simulink model "inverted"  (R2023b)
settings: Solver=VariableStepAuto  StartTime=0.0  StopTime=10.0  RelTol=1e-3
values from neighbouring files (symbols this model uses):
  A = [0 1 0 0 ... (first row only)    [invertedpendulum.m]
  B = [0 ... (first row only)    [invertedpendulum.m]
  C = [0 0 1 0]    [invertedpendulum.m]
  k = acker(A_bar,B_bar,cl_poles)    [invertedpendulum.m]
settings Model: Creator=mluser  LastModifiedBy=91798

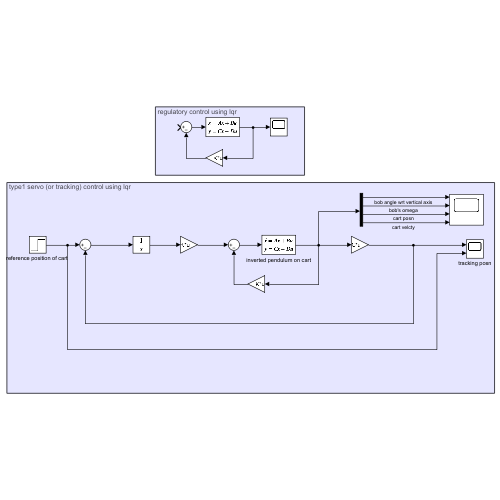
[thumbnail: Simulink's stored preview of the top-level diagram]
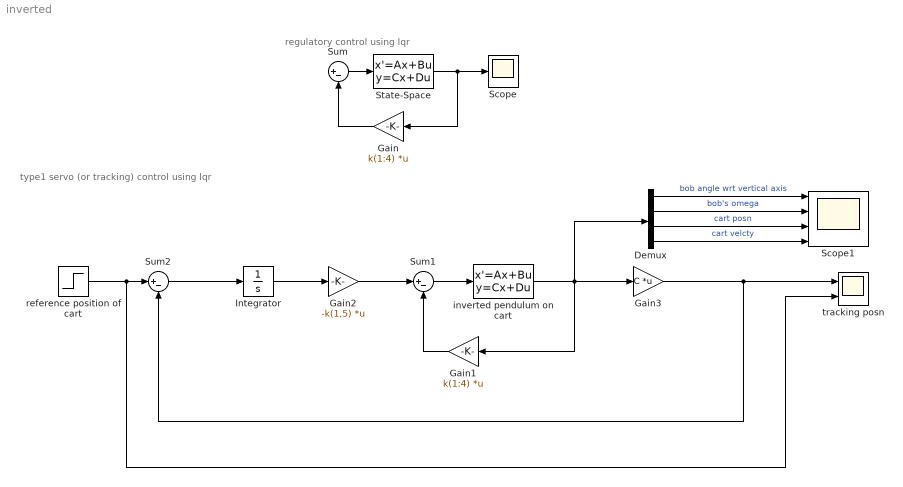
== system inverted ==
  note: type1 servo (or tracking) control using lqr
  note: regulatory control using lqr
  Demux : Demux
  Gain : Gain  Gain=k(1:4)  Multiplication=Matrix(K*u)
  Gain1 : Gain  Gain=k(1:4)  Multiplication=Matrix(K*u)
  Gain2 : Gain  Gain=-k(1,5)  Multiplication=Matrix(K*u)
  Gain3 : Gain  Gain=C  Multiplication=Matrix(K*u)
  Integrator : Integrator
  Scope : Scope
  Scope1 : Scope  NumInputPorts=4
  State-Space : StateSpace  A=A  B=B  C=eye(4)  D=zeros(4,1)  InitialCondition=[pi/6;0;0;0]
  Sum : Sum  Inputs=|+-
  Sum1 : Sum  Inputs=|+-
  Sum2 : Sum  Inputs=|+-
  inverted pendulum on cart : StateSpace  A=A  B=B  C=eye(4)  D=zeros(4,1)  InitialCondition=[0;1;2;3]
  "reference position of cart " : Step  Time=2  After=1.5  SampleTime=0
  tracking posn : Scope  NumInputPorts=2
  wires:
  Sum/1 -> State-Space/1
  State-Space/1 -> Scope/1, Gain/1
  Gain/1 -> Sum/2
  Gain1/1 -> Sum1/2
  inverted pendulum on cart/1 -> Demux/1, Gain3/1, Gain1/1
  Sum1/1 -> inverted pendulum on cart/1
  Integrator/1 -> Gain2/1
  Gain2/1 -> Sum1/1
  Gain3/1 -> Sum2/2, tracking posn/1
  Sum2/1 -> Integrator/1
  "reference position of cart "/1 -> Sum2/1, tracking posn/2
  Demux/1 -> Scope1/1  "bob angle wrt vertical axis"
  Demux/2 -> Scope1/2  "bob's omega"
  Demux/3 -> Scope1/3  "cart posn"
  Demux/4 -> Scope1/4  "cart velcty"
